simulink model "Control_Model"  (R2018a)
settings: Solver=FixedStepAuto  StartTime=0.0  StopTime=t_final  FixedStep=0.1  RelTol=1e-3
undefined symbols (not defined in the file or in its folder): eA, eB, eC, ex0, K
settings Model: Creator=Shouvik Chakraborty  LastModifiedBy=Shouvik Chakraborty

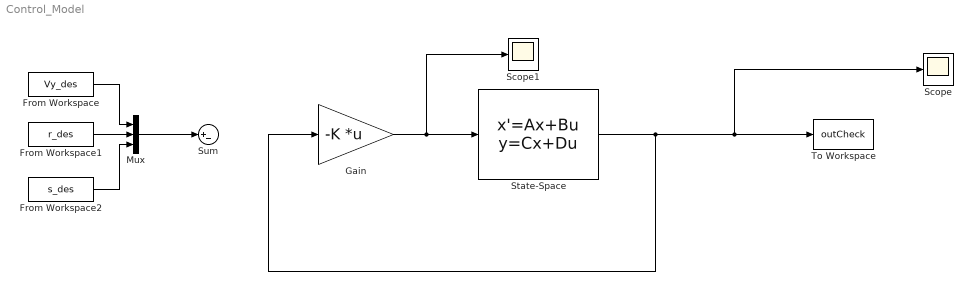
== system Control_Model ==
  From Workspace : FromWorkspace  VariableName=Vy_des  SampleTime=0
  From Workspace1 : FromWorkspace  VariableName=r_des  SampleTime=0
  From Workspace2 : FromWorkspace  VariableName=s_des  SampleTime=0
  Gain : Gain  Gain=-K  Multiplication=Matrix(K*u)
  Mux : Mux  Inputs=3
  Scope : Scope
  Scope1 : Scope
  State-Space : StateSpace  A=eA  B=eB  C=eC  D=[0;0;0;0;0]  InitialCondition=ex0
  Sum : Sum  Inputs=|+-
  To Workspace : ToWorkspace  VariableName=outCheck  SampleTime=-1
  wires:
  From Workspace1/1 -> Mux/2
  From Workspace/1 -> Mux/1
  From Workspace2/1 -> Mux/3
  Mux/1 -> Sum/1
  State-Space/1 -> Gain/1, Scope/1, To Workspace/1
  Gain/1 -> Scope1/1, State-Space/1
